simulink model "InsulationMeasurmentDevice"  (R2019b)
settings: Solver=FixedStepAuto  StartTime=0.0  StopTime=1.5  FixedStep=0.0004  RelTol=1e-3
libraries: pspsim x1
settings Model: Creator=ahmet  LastModifiedBy=ahmet
settings SFSimCC: SimCustomHeaderCode="#include \"insulation_monitor.h\""  SimUserSources=insulation_monitor.c

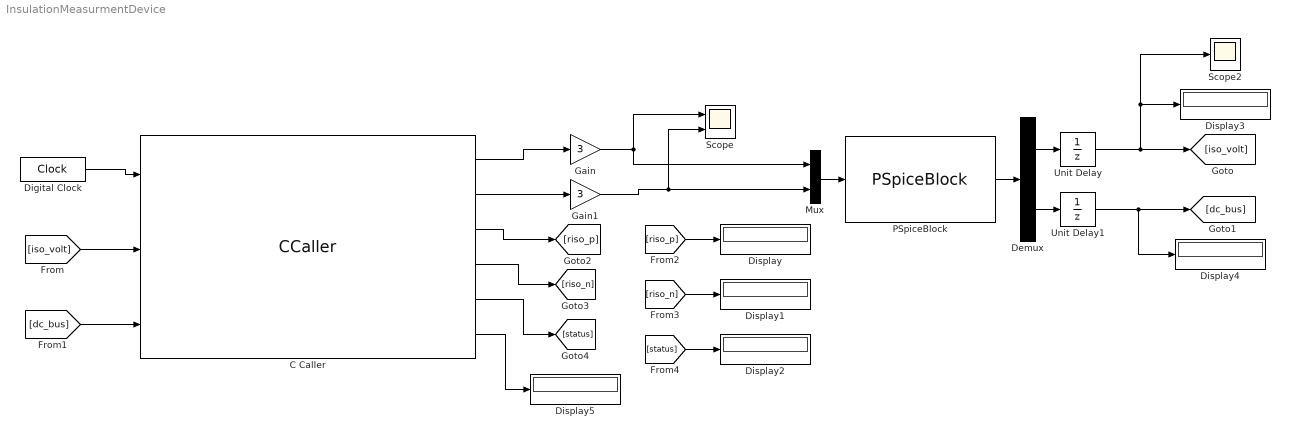
== system InsulationMeasurmentDevice ==
  C Caller : CCaller  FunctionName=insulation_measurement  PortSpecificationStruct="%)30     .    V \\   8    (     @         %    \"     D    !     0         %  0 \"0    $    _    07)G3F%M90  4&]R=$YA;64 4V-O<&4     26YD97@     5'EP90      4VEZ90      27-';&]B86P   X   !     !@    @    $          4    (     0    \\    !         !     /    <VEM=6QA=&EO;E]T:6UE  X   !     !@    @    $          4    (     0    \\    !         !     /    <VEM=6QA=&EO;E]T:6UE  X    X    !@    @    $  ...(+5099 chars)"
  Demux : Demux  Outputs=2
  Digital Clock : DigitalClock
  Display{,1..5} (6 alike) : Display
  Gain : Gain  Gain=3
  Gain1 : Gain  Gain=3
  Mux : Mux  Inputs=2
  PSpiceBlock : pspsim/PSpiceBlock  SFunctionModules=''
      settings: SourceProductName=PSpice Block
  Scope : Scope  NumInputPorts=2
  Scope2 : Scope
  Unit Delay : UnitDelay  SampleTime=-1  HasFrameUpgradeWarning=on
  Unit Delay1 : UnitDelay  SampleTime=-1  HasFrameUpgradeWarning=on
  wires:
  C Caller/5 -> [status]
  C Caller/4 -> [riso_n]
  C Caller/3 -> [riso_p]
  [riso_p] -> Display/1
  [riso_n] -> Display1/1
  [status] -> Display2/1
  C Caller/6 -> Display5/1
  C Caller/1 -> Gain/1
  C Caller/2 -> Gain1/1
  [dc_bus] -> C Caller/3
  [iso_volt] -> C Caller/2
  Digital Clock/1 -> C Caller/1
  Gain1/1 -> Mux/2, Scope/2
  PSpiceBlock/1 -> Demux/1
  Mux/1 -> PSpiceBlock/1
  Gain/1 -> Mux/1, Scope/1
  Demux/1 -> Unit Delay/1
  Demux/2 -> Unit Delay1/1
  Unit Delay/1 -> Scope2/1, Display3/1, [iso_volt]
  Unit Delay1/1 -> Display4/1, [dc_bus]
